simulink model "rrScenarioSimWithSensors - Copy"  (R2023b)
settings: Solver=FixedStepAuto  StartTime=0  StopTime=1000  FixedStep=simStepSize  RelTol=1e-3
undefined symbols (not defined in the file): Defined, driving, Ego, Lane, matlabshared, simStepSize, User
libraries: roadrunnerscenario x7, drivingscenarioandsensors x3
settings Model: Creator=The MathWorks, Inc.  LastModifiedBy=parks
settings DataIOCC: LimitDataPoints=on  MaxDataPoints=100  SaveFormat=StructureWithTime  SaveOutput=off  DSMLogging=off  DatasetSignalFormat=timetable
settings OptimizationCC: ReuseModelBlockBuffer=off
settings DebuggingCC: SubsystemReferenceDiagnosticForUnitTest=warning

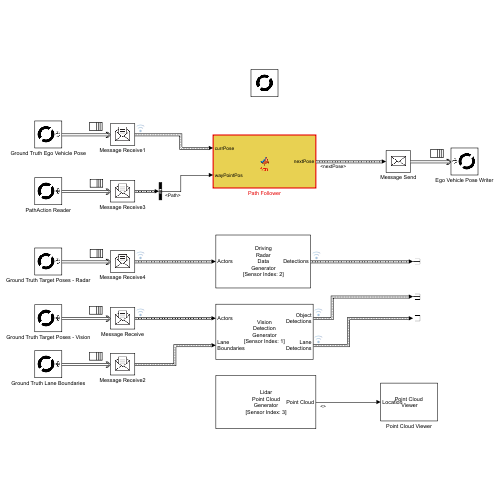
[thumbnail: Simulink's stored preview of the top-level diagram]
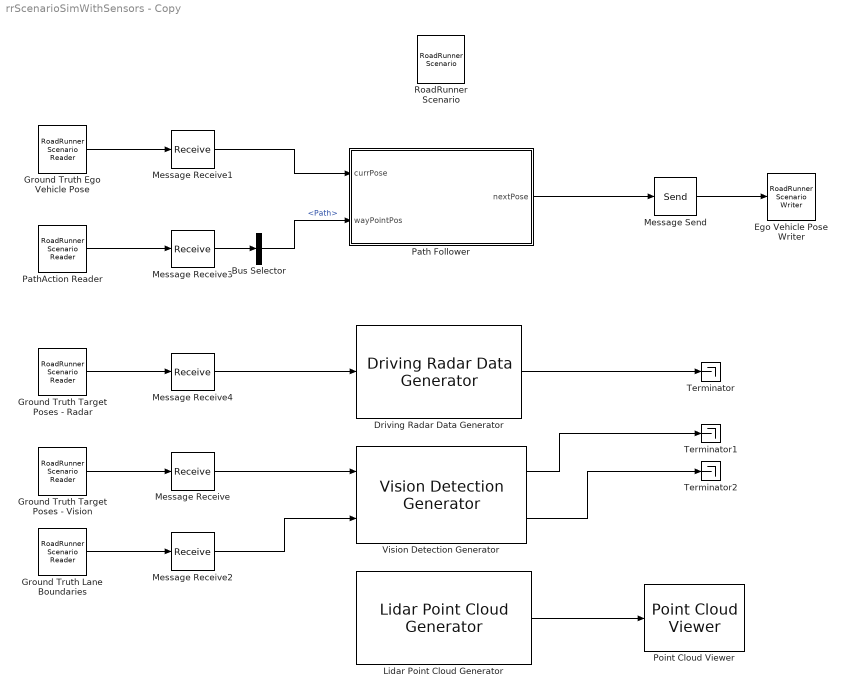
== system rrScenarioSimWithSensors - Copy ==
  Bus Selector : BusSelector  OutputSignals=PathTarget.Path
  Driving Radar Data Generator : drivingscenarioandsensors/Driving Radar Data Generator  SensorIndex=2  UpdateRate=1/simStepSize  MountingLocation=[1.8, 0, 0.2 ]  MountingAngles=[0 0 0]  HasElevation=off  HasRangeRate=on  HasNoise=on  HasFalseAlarms=on  HasOcclusion=on  MaxNumReportsSource=Property  MaxNumReports=50  TargetReportFormat=Detections  DetectionCoordinates=Body  TrackCoordinates=Body  BusNameSource=Auto  BusName=BusDrivingRadarDataGenerator  AzimuthResolution=1  ElevationResolution=5  RangeResolution=2.5  RangeRateResolution=0.5  AzimuthBiasFraction=0.1  ElevationBiasFraction=0.1  RangeBiasFraction=0.05  RangeRateBiasFraction=0.05  FieldOfView=[ 80, 5 ]  RangeLimits=[ 0, 150 ]  RangeRateLimits=[ -100, 100 ]  DetectionProbability=0.9  FalseAlarmRate=1e-06  ReferenceRange=100  ReferenceRCS=0  CenterFrequency=77e9  FilterInitializationFcn=initcvekf  ConfirmationThreshold=[2 3]  DeletionThreshold=[5 5]  InitialSeedSource=Repeatable  InitialSeed=0  UsedSeed=matlabshared.tracking.internal.SimulinkUtilities.seedManager(gcb)  ProfilesSource=From Scenario Reader block  ProfilesParameters=driving.internal.ActorProfilesRadarParameters  ProfilesExpression=struct('ClassID',0,'Length',4.7,'Width',1.8,'Height',1.4,'OriginOffset',[-1.35 0 0],'RCSPattern',[10 10;10 10],'RCSAzimuthAngles',[-180 180],'RCSElevationAngles',[-90 90])
  Ego Vehicle Pose Writer : roadrunnerscenario/RoadRunner Scenario Writer  TopicCategory=Actor  ActorCategory=All Types  EventType=Action Complete  UserDefinedEvent=Event1  VehicleType=Vehicle Pose  TopicType=Actor Pose
  Ground Truth Ego Vehicle Pose : roadrunnerscenario/RoadRunner Scenario Reader  TopicCategory=Actor  ActorCategory=All Types  ActionType=Path Following  EventType=User-Defined  TopicType=Actor Pose  VehicleType=Vehicle Pose  UserDefinedAction=Action1  UserDefinedEvent=Event1  Filter=Self  SensorTopic=Target Poses  LaneBoundaryOutputTopic=Ego-Lane  SensorID=1  SampleTime=simStepSize
  Ground Truth Lane Boundaries : roadrunnerscenario/RoadRunner Scenario Reader  TopicCategory=Sensor  ActorCategory=All Types  ActionType=Path Following  EventType=User-Defined  TopicType=Actor Pose  VehicleType=Vehicle Pose  UserDefinedAction=Action1  UserDefinedEvent=Event1  Filter=Self  SensorTopic=Lane Boundaries  LaneBoundaryOutputTopic=Ego and Adjacent Lanes  SensorID=1  SampleTime=simStepSize
  Ground Truth Target Poses - Radar : roadrunnerscenario/RoadRunner Scenario Reader  TopicCategory=Sensor  ActorCategory=All Types  ActionType=Path Following  EventType=User-Defined  TopicType=Actor Specifications  VehicleType=Vehicle Specifications  UserDefinedAction=Action1  UserDefinedEvent=Event1  Filter=Self  SensorTopic=Target Poses  LaneBoundaryOutputTopic=Ego-Lane  SensorID=2  SampleTime=simStepSize
  Ground Truth Target Poses - Vision : roadrunnerscenario/RoadRunner Scenario Reader  TopicCategory=Sensor  ActorCategory=All Types  ActionType=Path Following  EventType=User-Defined  TopicType=Actor Specifications  VehicleType=Vehicle Specifications  UserDefinedAction=Action1  UserDefinedEvent=Event1  Filter=Self  SensorTopic=Target Poses  LaneBoundaryOutputTopic=Ego-Lane  SensorID=1  SampleTime=simStepSize
  Lidar Point Cloud Generator : drivingscenarioandsensors/Lidar Point Cloud Generator  SensorIndex=3  UpdateInterval=simStepSize  SensorLocation=[1.5 0]  Height=1.6  Yaw=0  Pitch=0  Roll=0  DetectionCoordinates=Ego Cartesian  HasEgoVehicle=on  EgoVehicleActorID=1  HasRoadsInputPort=on  ActorProfilesSource=From Scenario Reader block  ActorProfilesVariableName=actor_profiles  MaxRange=120  RangeAccuracy=0.002  AzimuthResolution=0.16  ElevationResolution=1.25  AzimuthLimits=[ -180, 180 ]  ElevationLimits=[ -20, 20 ]  HasNoise=on
  Message Receive{,1..4} (5 alike) : Receive  InputPortMessageModes=m  UseInternalQueue=off  SampleTime=simStepSize
  Message Send : Send  OutputPortMessageModes=m
  Path Follower : MATLAB Function  TreatAsAtomicUnit=on
  PathAction Reader : roadrunnerscenario/RoadRunner Scenario Reader  TopicCategory=Action  ActorCategory=All Types  ActionType=Path Following  EventType=User-Defined  TopicType=Actor Specifications  VehicleType=Vehicle Specifications  UserDefinedAction=Action1  UserDefinedEvent=Event1  Filter=Self  SensorTopic=Target Poses  LaneBoundaryOutputTopic=Ego-Lane  SensorID=1  SampleTime=simStepSize
  Point Cloud Viewer : PointCloudViewer  FigPos=[1096.33333333333 439.333333333333 410 300]
  RoadRunner Scenario : roadrunnerscenario/RoadRunner Scenario  UserDefinedActions={}  UserDefinedEvents={}
  Terminator : Terminator
  Terminator1 : Terminator
  Terminator2 : Terminator
  Vision Detection Generator : drivingscenarioandsensors/Vision Detection Generator  SensorIndex=1  DetectorOutput=Lanes and objects  UpdateInterval=simStepSize  LaneUpdateInterval=simStepSize  SensorLocation=[1.2 0]  Height=1.1  Yaw=0  Pitch=1  Roll=0  BusNameSource=Auto  BusName=BusObjectDetections  BusName2Source=Auto  BusName2=BusLaneDetections  MaxNumDetectionsSource=Property  MaxNumDetections=50  MaxNumLanesSource=Property  MaxNumLanes=30  DetectionCoordinates=Ego Cartesian  SimulateUsing=Interpreted execution  MaxRange=150  BoundingBoxAccuracy=5  ProcessNoiseIntensity=5  MaxSpeed=100  MaxAllowedOcclusion=0.5  MinObjectImageSize=[ 15, 15 ]  DetectionProbability=0.9  FalsePositivesPerImage=0.1  MinLaneImageSize=[ 20, 3 ]  LaneBoundaryAccuracy=3  HasNoise=on  InitialSeedSource=Repeatable  InitialSeed=0  UsedSeed=driving.internal.SimulinkUtilities.seedManager(gcb)  ActorProfilesSource=From Scenario Reader block  ActorProfilesParameters=driving.internal.ActorProfilesParameters  ActorProfilesExpression=actorProfiles  Intrinsics=driving.internal.cameraIntrinsics('FocalLength',[ 1200, 1200 ])
  wires:
  Ground Truth Target Poses - Vision/1 -> Message Receive/1
  Vision Detection Generator/1 -> Terminator1/1
  Message Receive/1 -> Vision Detection Generator/1
  Ground Truth Ego Vehicle Pose/1 -> Message Receive1/1
  Path Follower/1(nextPose) -> Message Send/1
  Message Receive1/1 -> Path Follower/1(currPose)
  PathAction Reader/1 -> Message Receive3/1
  Message Receive3/1 -> Bus Selector/1
  Message Send/1 -> Ego Vehicle Pose Writer/1
  Bus Selector/1 -> Path Follower/2(wayPointPos)  "<Path>"
  Ground Truth Lane Boundaries/1 -> Message Receive2/1
  Message Receive2/1 -> Vision Detection Generator/2
  Vision Detection Generator/2 -> Terminator2/1
  Driving Radar Data Generator/1 -> Terminator/1
  Ground Truth Target Poses - Radar/1 -> Message Receive4/1
  Message Receive4/1 -> Driving Radar Data Generator/1
  Lidar Point Cloud Generator/1 -> Point Cloud Viewer/1

== matlab function rrScenarioSimWithSensors - Copy/Path Follower ==
  data: currPose input; wayPointPos input; nextPose output Bus: BusActorRuntime; simStepSize parameter
function nextPose  = fcn(currPose, wayPointPos,simStepSize)

% Set constant ego vehicle speed
egoSpeed  = 18;

% Declare persistent variables for simulation and retain only non zero
% elements in the array of waypoints 
persistent wayPointIdx wayPointPosInterp headingAnglesInterp numWayPoints
wayPointPos = reshape(wayPointPos(wayPointPos~=0),[],2);

% Extract poses for the entire path before simulation begins
if isempty(wayPointIdx)
    
    wayPointIdx = 2;

    % Pre-allocate arrays
    numInputPoints = length(wayPointPos);
    trueTimes = zeros(numInputPoints+1,1);
    headingAngles = zeros(numInputPoints,1);
    wayPointPosInterp = [];
    headingAnglesInterp = [];

    startPoint = [currPose.Pose(1,4) currPose.Pose(2,4)];
    currPoint = startPoint;

    % Loop through all the input points
    for i=1:numInputPoints

        % Calculate distance from the current point to the next point
        nextPoint = wayPointPos(i,1:2);
        delXY = nextPoint-currPoint;
        absDistToNextPoint = norm(delXY);
        
        % Calculate time of arrival at the next wayPoint based on the
        % set constant speed. Alternatively, you can set the timing profile
        % in RoadRunner for waypoints and use those here 
        trueTimes(i+1) = absDistToNextPoint/egoSpeed + trueTimes(i);
        
        % Calculate the heading angle to proceed towards the next waypoint
        headingAngles(i) = atan2d(delXY(2),delXY(1))-90;
        
        % Based on the simulation step size, calculate the time vector
        % between arrival times at previous waypoint and the current waypoint
        tvec = trueTimes(i):simStepSize:trueTimes(i+1);
        
        % Interpolate X and Y positions between the current and next waypoints
        % along the entire time vector. Store them
        interpPosPointsX = interp1(linspace(trueTimes(i),trueTimes(i+1),100),...
                linspace(currPoint(1),nextPoint(1),100),...
                tvec)';
    
        interpPosPointsY = interp1(linspace(trueTimes(i),trueTimes(i+1),100),...
                linspace(currPoint(2),nextPoint(2),100),...
                tvec)';
        
        wayPointPosInterp = [wayPointPosInterp;[interpPosPointsX interpPosPointsY]];

        % Use the constant heading angle towards the next waypoint for all
        % interpolated points between them
        headingAnglesInterp = [headingAnglesInterp;headingAngles(i)*ones(size(interpPosPointsX))];

        currPoint = nextPoint;
    end

    % Get the new total number of waypoints after interpolation
    numWayPoints = length(wayPointPosInterp);
end

% At each time step of the simulation, send the next waypoint position from the
% interpolated waypoint array until ego vehicle arrives at the last waypoint
nextPose = currPose;
nextPose.Pose(1,4) = wayPointPosInterp(wayPointIdx,1);
nextPose.Pose(2,4) = wayPointPosInterp(wayPointIdx,2);

% Convert the heading angle (yaw) to a rotation matrix
nextPose.Pose(1:3,1:3) = [cosd(headingAnglesInterp(wayPointIdx)) -sind(headingAnglesInterp(wayPointIdx)) 0;...
                          sind(headingAnglesInterp(wayPointIdx)) cosd(headingAnglesInterp(wayPointIdx)) 0;...
                          0 0 1];

if(wayPointIdx<numWayPoints)
    wayPointIdx = wayPointIdx + 1;
end

end
